simulink model "Pr3"  (R2022b)
settings: Solver=ode23  StartTime=0.0  StopTime=50  RelTol=1e-3
settings Model: Creator=rus_d  LastModifiedBy=rus_d

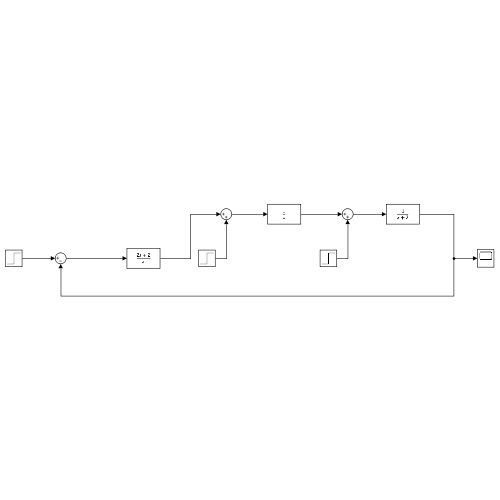
[thumbnail: Simulink's stored preview of the top-level diagram]
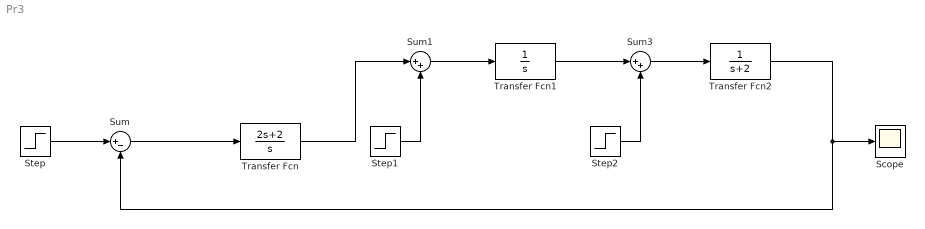
== system Pr3 ==
  Scope : Scope
  Step : Step  SampleTime=0
  Step1 : Step  Time=25  After=0.2  SampleTime=0
  Step2 : Step  Time=40  After=0.5  SampleTime=0
  Sum : Sum  Inputs=|+-
  Sum1 : Sum  Inputs=|++
  Sum3 : Sum  Inputs=|++
  Transfer Fcn : TransferFcn  Numerator=[2 2 ]  Denominator=[1 0]
  Transfer Fcn1 : TransferFcn  Denominator=[1 0]
  Transfer Fcn2 : TransferFcn  Denominator=[1 2]
  wires:
  Step1/1 -> Sum1/2
  Sum1/1 -> Transfer Fcn1/1
  Step/1 -> Sum/1
  Transfer Fcn/1 -> Sum1/1
  Sum/1 -> Transfer Fcn/1
  Transfer Fcn2/1 -> Sum/2, Scope/1
  Step2/1 -> Sum3/2
  Transfer Fcn1/1 -> Sum3/1
  Sum3/1 -> Transfer Fcn2/1
